simulink model "Task_1E"  (R2022a)
settings: Solver=VariableStepAuto  StartTime=0.0  StopTime=50  RelTol=1e-3
values from neighbouring files (symbols this model uses):
  d_COM = R_robot * cos(theta_wheels)    [Parameter_Setup.m]
  L_wheel = R_robot * sin(theta_wheels)    [Parameter_Setup.m]
  m_total = m_load + m_robot    (= 40)    [Parameter_Setup.m]
  R_wheel = D_wheel/2    (= 0.05)    [Parameter_Setup.m]
settings Model: Creator=jpcas  LastModifiedBy=jpcas

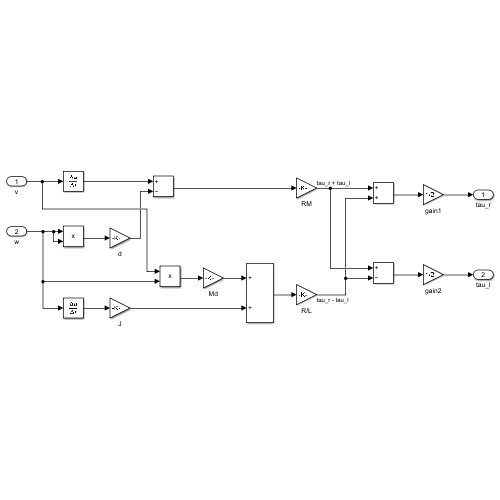
[thumbnail: Simulink's stored preview of the top-level diagram]
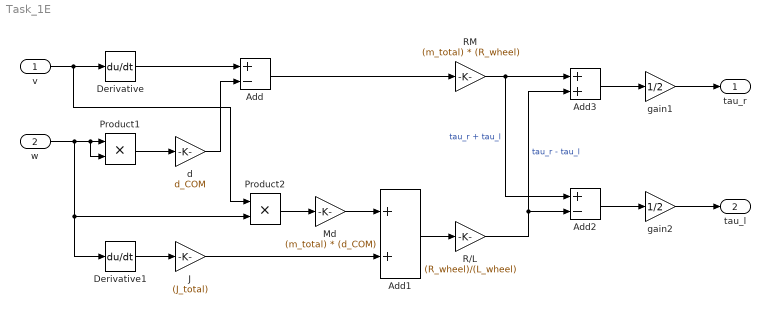
== system Task_1E ==
  v : Inport
  w : Inport  Port=2
  Add : Sum  Inputs=+-
  Add1 : Sum
  Add2 : Sum  Inputs=+-
  Add3 : Sum
  Derivative : Derivative
  Derivative1 : Derivative
  J : Gain  Gain=(J_total)
  Md : Gain  Gain=(m_total) * (d_COM)
  Product1 : Product
  Product2 : Product
  R/L : Gain  Gain=(R_wheel)/(L_wheel)
  RM : Gain  Gain=(m_total) * (R_wheel)
  d : Gain  Gain=d_COM
  gain1 : Gain  Gain=1/2
  gain2 : Gain  Gain=1/2
  tau_r : Outport
  tau_l : Outport  Port=2
  wires:
  v/1 -> Product2/1, Derivative/1
  Product1/1 -> d/1
  w/1 -> Product2/2, Derivative1/1, Product1/1, Product1/2
  Derivative/1 -> Add/1
  d/1 -> Add/2
  Add/1 -> RM/1
  Derivative1/1 -> J/1
  Product2/1 -> Md/1
  J/1 -> Add1/2
  Md/1 -> Add1/1
  Add1/1 -> R/L/1
  RM/1 -> Add2/1, Add3/1  "tau_r + tau_l"
  R/L/1 -> Add2/2, Add3/2  "tau_r - tau_l"
  Add3/1 -> gain1/1
  Add2/1 -> gain2/1
  gain1/1 -> tau_r/1
  gain2/1 -> tau_l/1
